simulink model "MPC_unconstrained"  (R2024a)
settings: Solver=VariableStepAuto  StartTime=0.0  StopTime=10.0  RelTol=1e-3
values from neighbouring files (symbols this model uses):
  N = 5    [project_script.m]    (also in scriptpoint7.m)
  Qd = 10*eye(2)    [project_script.m]    (also in scriptpoint7.m = 1000*eye(2))
  Rd = 1*eye(2)    [project_script.m]    (also in scriptpoint7.m)
  S0 = zeros(2)    [project_script.m]    (also in scriptpoint7.m)
  Ts = 1/8000    (= 0.000125)    [project_script.m]    (also in scriptpoint7.m)
  u_bar_d = Bd\ (eye(size(Ad))-Ad)*xref    [project_script.m]    (also in scriptpoint7.m)
  u_sat_max = [u1_max; u2_max]    [project_script.m]    (also in scriptpoint7.m)
  u_sat_min = [u1_min; u2_min]    [project_script.m]    (also in scriptpoint7.m)
  x0 = [x0_1;x0_2]    [project_script.m]    (also in scriptpoint7.m)
  x_sat_max = [x1_max; x2_max]    [project_script.m]    (also in scriptpoint7.m)
  x_sat_min = [x1_min; x2_min]    [project_script.m]    (also in scriptpoint7.m)
  xref = [6.9; 8.9]    [project_script.m]    (also in scriptpoint7.m)
undefined symbols (not defined in the file or in its folder): Ad, Bd, Cd, Dd, mympc
settings Model: Creator=Utente  LastModifiedBy=papidrago

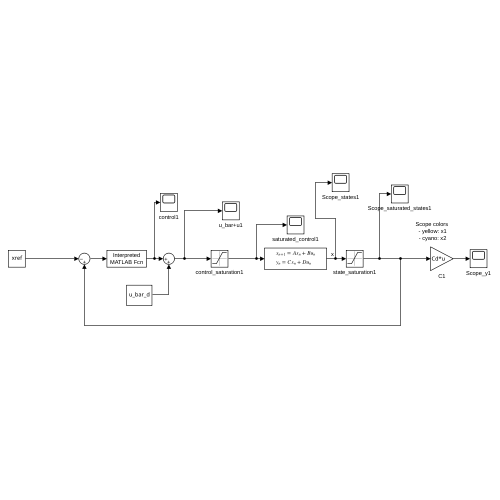
[thumbnail: Simulink's stored preview of the top-level diagram]
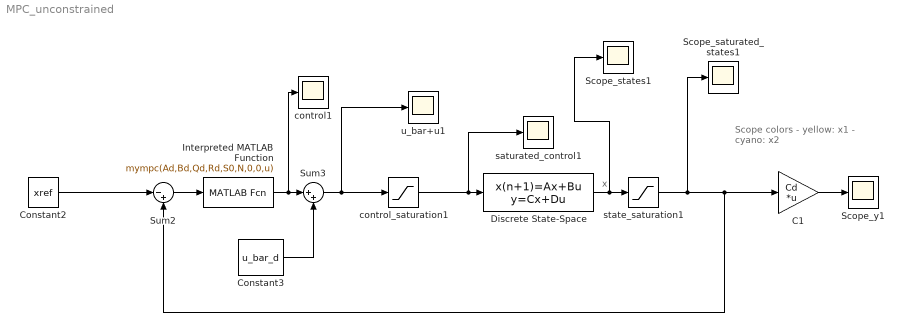
== system MPC_unconstrained ==
  note: x
  note: Scope colors
      | - yellow: x1
      | - cyano: x2
  C1 : Gain  Gain=Cd  Multiplication=Matrix(K*u)
  Constant2 : Constant  Value=xref  SampleTime=Ts
  Constant3 : Constant  Value=u_bar_d  SampleTime=Ts
  Discrete State-Space : DiscreteStateSpace  A=Ad  B=Bd  C=Cd  D=Dd  InitialCondition=x0  SampleTime=Ts
  Interpreted MATLAB Function : MATLABFcn  MATLABFcn=mympc(Ad,Bd,Qd,Rd,S0,N,0,0,u)
  Scope_saturated_states1 : Scope
  Scope_states1 : Scope
  Scope_y1 : Scope
  Sum2 : Sum  Inputs=|-+
  Sum3 : Sum  Inputs=|++
  control1 : Scope
  control_saturation1 : Saturate  UpperLimit=u_sat_max  LowerLimit=u_sat_min
  saturated_control1 : Scope
  state_saturation1 : Saturate  UpperLimit=x_sat_max  LowerLimit=x_sat_min
  u_bar+u1 : Scope
  wires:
  Sum3/1 -> control_saturation1/1, u_bar+u1/1
  control_saturation1/1 -> saturated_control1/1, Discrete State-Space/1
  C1/1 -> Scope_y1/1
  Constant2/1 -> Sum2/1
  Discrete State-Space/1 -> Scope_states1/1, state_saturation1/1
  Constant3/1 -> Sum3/2
  state_saturation1/1 -> Sum2/2, C1/1, Scope_saturated_states1/1
  Sum2/1 -> Interpreted MATLAB Function/1
  Interpreted MATLAB Function/1 -> control1/1, Sum3/1
